simulink model "Robo_Bipede_Contato"  (R2020a)
settings: Solver=ode15s  StartTime=0.0  StopTime=1  MaxStep=1e-4  RelTol=1e-4  AbsTol=1e-5  EnableMultiTasking=on
model workspace: external: MATLAB File C:\Users\LUIS IZQUIERDO C\Desktop\PROGRAMAS TESE\13. ROBO BIPEDE SIMSCAPE COM CONTATO\Model_Params_Contato.m (data not in the file)
values from neighbouring files (symbols this model uses):
  CoG_y = 0.091733    [Model_Params_Cont_FSM.m]
  height_plane = 0.025    [Model_Params_Cont_FSM.m]
  m_esfera = 1    [Model_Params_Cont_FSM.m]
  plane_height = height_plane    (= 0.025)    [Model_Params_Cont_FSM.m]
  plane_length = 50    [Model_Params_Cont_FSM.m]
  plane_width = 3    [Model_Params_Cont_FSM.m]
  temp = Dados_XY1_D(ciclo,1)    [Model_Params_Cont_FSM.m]
  velocidade = 1    [Model_Params_Cont_FSM.m]
  Xpq2_D = Xpq2_D'    [Model_Params_Cont_FSM.m]
  Xpq3_D = Xpq3_D'    [Model_Params_Cont_FSM.m]
  Ypq2_D = Ypq2_D'    [Model_Params_Cont_FSM.m]
  Ypq3_D = Ypq3_D'    [Model_Params_Cont_FSM.m]
undefined symbols (not defined in the file or in its folder): COXA, HAT, PE, PERNA, X, Y, Z
libraries: nesl_utility x70, sm_lib x61, simulink x1
(part 1 of 3)
settings Model: Creator=LUIS IZQUIERDO C  LastModifiedBy=LUIS IZQUIERDO C
settings DataIOCC: LimitDataPoints=on  ReturnWorkspaceOutputs=off  LoggingToFile=on
settings OptimizationCC: LifeSpan=inf
settings DebuggingCC: AllowSymbolicDim=off  SFUnexpectedBacktrackingDiag=warning  SFNoUnconditionalDefaultTransitionDiag=warning  SFExecutionAtInitializationDiag=none  ArithmeticOperatorsInVariantConditions=warning
settings SFSimCC: SimUseLocalCustomCode=off  CustomCodeUndefinedFunction=UseInterfaceOnly
settings RTWCC: RTWUseLocalCustomCode=off
settings CodeAppCC: StateflowObjectComments=on
settings GRTTargetCC: TargetLangStandard=C89/C90 (ANSI)
settings ConfigComp: CovMetricSettings=dw  CovHtmlReporting=on  CovSaveCumulativeToWorkspaceVar=on  CovSaveSingleToWorkspaceVar=on  CovExternalEMLEnable=off  CovSFcnEnable=off
settings SimscapeCC: SimscapeNominalValues="[{\"value\":\"10\",\"unit\":\"V\"},{\"value\":\"1\",\"unit\":\"A\"},{\"value\":\"10\",\"unit\":\"N*m\"},{\"value\":\"10\",\"unit\":\"bar\"},{\"value\":\"100\",\"unit\":\"kJ/kg\"},{\"value\":\"1\",\"unit\":\"kW\"},{\"value\":\"300\",\"unit\":\"K\"},{\"value\":\"100\",\"unit\":\"cm^3/s\"},{\"value\":\"1\",\"unit\":\"kN\"},{\"value\":\"1\",\"unit\":\"g/cm^3\"},{\"value\":\"1\",\"unit\":\"l\"},{\"value\":\"1\",\"unit\":\"cm^2\"},{\"value\":\"60\",\"unit\":\"Hz\"}]"  SimscapeLogType=all  SimscapeLogDataHistory=10000
settings ConfigurationSet: Description=SimMechanics 2G

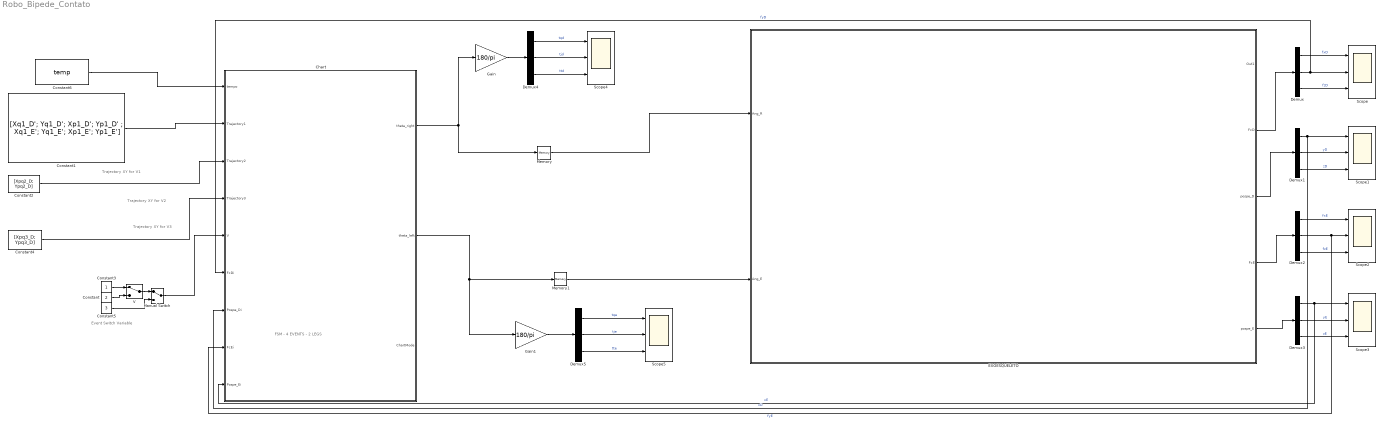
== system Robo_Bipede_Contato ==
  note: Trajectory XY for V1
  note: FSM - 4 EVENTS - 2 LEGS
  note: Trajectory XY for V2
  note: Trajectory XY for V3
  note: Event Switch Variable
  Chart : Stateflow chart  TreatAsAtomicUnit=on
  Constant : Constant  Value=2
  Constant1 : Constant  Value=|  VectorParams1D=off
      | [Xq1_D'; Yq1_D'; Xp1_D';
      | Yp1_D'
      | ;  Xq1_E';
      | Yq1_E';
      | Xp1_E';
      | Yp1_E']
  Constant2 : Constant  Value=[Xpq2_D; Ypq2_D]  VectorParams1D=off
  Constant3 : Constant
  Constant4 : Constant  Value=[Xpq3_D; Ypq3_D]  VectorParams1D=off
  Constant5 : Constant  Value=3
  Constant6 : Constant  Value=temp  VectorParams1D=off
  Demux{,1..5} (6 alike) : Demux  Outputs=3
  EXOESQUELETO : Subsystem
  Gain : Gain  Gain=180/pi
  Gain1 : Gain  Gain=180/pi
  Manual Switch : ManualSwitch
  Memory : Memory
  Memory1 : Memory
  Scope{,1..5} (6 alike) : Scope  NumInputPorts=3
  V : ManualSwitch
  wires:
  EXOESQUELETO/5(pospe_E) -> Demux3/1
  EXOESQUELETO/2(FcD) -> Demux/1
  Demux/1 -> Scope/1  "fxD"
  Demux/2 -> Chart/6(FcDi), Scope/2  "fyD"
  Demux/3 -> Scope/3  "fzD"
  Demux1/1 -> Chart/7(Pospe_Di), Scope1/1  "xD"
  Demux1/2 -> Scope1/2  "yD"
  Demux1/3 -> Scope1/3  "zD"
  Demux3/1 -> Chart/9(Pospe_Ei), Scope3/1  "xE"
  Demux3/2 -> Scope3/2  "yE"
  Demux2/1 -> Scope2/1  "fxE"
  Demux2/2 -> Chart/8(FcEi), Scope2/2  "fyE"
  Demux2/3 -> Scope2/3  "fzE"
  Demux3/3 -> Scope3/3  "zE"
  EXOESQUELETO/3(pospe_D) -> Demux1/1
  EXOESQUELETO/4(FcE) -> Demux2/1
  Constant3/1 -> V/1
  V/1 -> Manual Switch/1
  Manual Switch/1 -> Chart/5(V)
  Constant2/1 -> Chart/3(Trajectory2)
  Constant/1 -> V/2
  Constant4/1 -> Chart/4(Trajectory3)
  Constant5/1 -> Manual Switch/2
  Constant1/1 -> Chart/2(Trajectory1)
  Constant6/1 -> Chart/1(tempo)
  Chart/1(theta_right) -> Memory/1, Gain/1
  Memory/1 -> EXOESQUELETO/1(Ang_R)
  Memory1/1 -> EXOESQUELETO/2(Ang_E)
  Chart/2(theta_left) -> Gain1/1, Memory1/1
  Demux5/1 -> Scope5/1  "tqe"
  Demux5/2 -> Scope5/2  "tje"
  Demux5/3 -> Scope5/3  "tte"
  Demux4/2 -> Scope4/2  "tjd"
  Demux4/1 -> Scope4/1  "tqd"
  Demux4/3 -> Scope4/3  "ttd"
  Gain/1 -> Demux4/1
  Gain1/1 -> Demux5/1

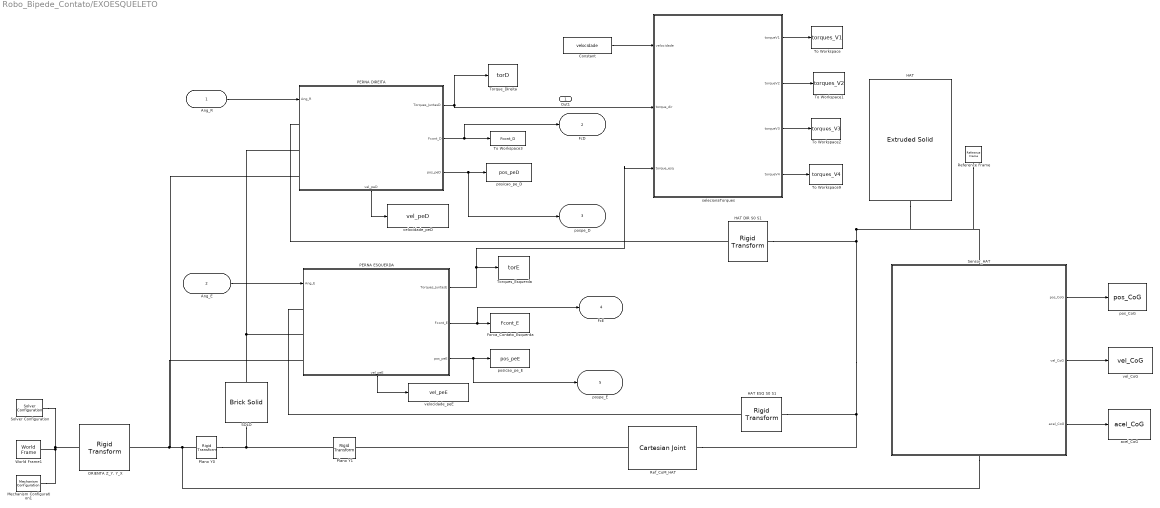
== system Robo_Bipede_Contato/EXOESQUELETO ==
  Ang_R : Inport
  Ang_E : Inport  Port=2
  Constant : Constant  Value=velocidade
  Forca_Contato_Esquerda : ToWorkspace  VariableName=Fcont_E  SaveFormat=Timeseries  SampleTime=-1
  HAT : sm_lib/Body Elements/Extruded Solid  GraphicAmbientColor=[0.15 0.15 0.15 1.0]  BasedOnType=Density  CenterOfMass=[0 0 0]  CenterOfMassUnits=m  GraphicDiffuseColor=[0.9 0.5 0.5]  ExportConvexHullGeometry=off  ExtrusionCrossSection=hat_cross_sec  ExtrusionCrossSectionUnits=m  Density=rho_ABS  DensityUnits=kg/m^3  DoExposeReferenceFrame=off  GraphicEmissiveColor=[0.0 0.0 0.0 1.0]  ExportEntireGeometry=off  ExtrusionLength=HAT.Profundidade  ExtrusionLengthUnits=m  ExtrusionType=General  SerializedFrames=<Frames><Frame><Id>Frame1</Id><Value><Name>CoG</Name><Origin><Source>CenterOfMassFrame</Source><FeatureName></FeatureName></Origin><PrimaryAxis><DefinedDirection>+Y</DefinedDirection><Source>CenterOfMassFrame</Source><SourceDirection>+Y</SourceDirection><FeatureName></FeatureName></PrimaryAxis><SecondaryAxis><DefinedDirection>+X</DefinedDirection><Source>CenterOfMassFrame</Source><SourceDirection>+Z</SourceDirection><FeatureName></FeatureName></SecondaryAxis></Value></Frame></Frames>  MarkerShape=Sphere  MarkerSize=10  GraphicType=FromGeometry  InertiaType=CalculateFromGeometry  Mass=HAT.Massa  MassUnits=kg  MomentsOfInertia=[1 1 1]  MomentsOfInertiaUnits=kg*m^2  PolygonNumSides=3  GraphicOpacity=1.0  PolygonOuterRadius=1  PolygonOuterRadiusUnits=m  ProductsOfInertia=[0 0 0]  ProductsOfInertiaUnits=kg*m^2  GraphicShininess=75  GraphicSpecularColor=[0.5 0.5 0.5 1.0]  GraphicVisPropType=SimpleVisualProperties
  HAT DIR S0 S1 : sm_lib/Frames and Transforms/Rigid Transform  TranslationMethod=Cartesian  TranslationStandardOffset=0  TranslationLengthUnit=m  TranslationStandardAxis=+Z  TranslationCartesianOffset="[0, -CoG_y,  HAT.Largura/2]"  TranslationROffset=0  TranslationROffsetUnits=m  TranslationZOffset=0  TranslationZOffsetUnits=m  TranslationThetaOffset=0  TranslationThetaOffsetUnits=deg  RotationMethod=None  RotationAngleUnits=deg  RotationStandardAxis=+Z  RotationAngle=0.0  RotationArbitraryAxis=[0 0 1]  FollAlignAxisA=+X  BaseAlignAxisA=+Y  FollAlignAxisB=+Y  BaseAlignAxisB=+Z  RotationSequenceAxes=FollowerAxes  RotationSequence=XYX  RotationSequenceAngles=[0 0 0]  RotationSequenceAnglesUnits=deg  RotationMatrix=[1 0 0; 0 1 0; 0 0 1]
  HAT ESQ S0 S1 : sm_lib/Frames and Transforms/Rigid Transform  TranslationMethod=Cartesian  TranslationStandardOffset=0  TranslationLengthUnit=m  TranslationStandardAxis=+Z  TranslationCartesianOffset="[0, -CoG_y,  -HAT.Largura/2]"  TranslationROffset=0  TranslationROffsetUnits=m  TranslationZOffset=0  TranslationZOffsetUnits=m  TranslationThetaOffset=0  TranslationThetaOffsetUnits=deg  RotationMethod=None  RotationAngleUnits=deg  RotationStandardAxis=+Z  RotationAngle=0.0  RotationArbitraryAxis=[0 0 1]  FollAlignAxisA=+X  BaseAlignAxisA=+Y  FollAlignAxisB=+Y  BaseAlignAxisB=+Z  RotationSequenceAxes=FollowerAxes  RotationSequence=XYX  RotationSequenceAngles=[0 0 0]  RotationSequenceAnglesUnits=deg  RotationMatrix=[1 0 0; 0 1 0; 0 0 1]
  Mechanism Configuration1 : sm_lib/Utilities/Mechanism Configuration  UniformGravity=Constant  GravityVector="[0, 0, -9.80665  ]"  GravityUnits=m/s^2  LinearizationDelta=0.001
  "ORIENTA Z_Y, Y_X " : sm_lib/Frames and Transforms/Rigid Transform  TranslationMethod=None  TranslationStandardOffset=0  TranslationLengthUnit=m  TranslationStandardAxis=+Z  TranslationCartesianOffset=[0 0 0]  TranslationROffset=0  TranslationROffsetUnits=m  TranslationZOffset=0  TranslationZOffsetUnits=m  TranslationThetaOffset=0  TranslationThetaOffsetUnits=deg  RotationMethod=AlignedAxes  RotationAngleUnits=deg  RotationStandardAxis=+Z  RotationAngle=0.0  RotationArbitraryAxis=[0 0 1]  FollAlignAxisA=+Y  BaseAlignAxisA=+Z  FollAlignAxisB=+X  BaseAlignAxisB=+Y  RotationSequenceAxes=FollowerAxes  RotationSequence=XYX  RotationSequenceAngles=[0 0 0]  RotationSequenceAnglesUnits=deg  RotationMatrix=[1 0 0; 0 1 0; 0 0 1]
  PERNA DIREITA : Subsystem
      settings: PortSchema="{\"entries\":[{\"content\":{\"sides\":[{\"content\":{\"connectorIds\":[\"In1\",\"LConn1\",\"LConn2\",\"LConn3\"]},\"type\":\"ConnectorPlacement.EquallySpacedRectSide\",\"uuid\":\"cc7b771d-19b2-48a5-9b25-497eb2125d6a\"},{\"content\":{\"connectorIds\":[\"Out1\",\"Out2\",\"Out3\"],\"side\":\"RIGHT\"},\"type\":\"ConnectorPlacement.EquallySpacedRectSide\",\"uuid\":\"a76f2280-f57a-4bff-8789-f2695d488ae9\"},{\"content\":{\"connectorIds\":[],\"side\":\"TOP\"},\"type\":\"ConnectorPlacement.EquallySpacedRectSide\",\"uuid\":\"65c05dcd-433d-4d8c-b019-0656464b6d1d\"},{\"content\":{\"connectorIds\":[\"Out4\"],\"side\":\"BOTTOM\"},\"type\":\"ConnectorPlacement.EquallySpacedRectSide\",\"uuid\":\"da520478-eb90-4d51-a918-9a7423737d50\"}]},\"type\":\"ConnectorPlacement.EquallySpacedConnector\",\"uuid\":\"0c78c314-db55-406a-a70d-77132cc9a0df\"}],\"packageUris\":[\"http://schema.mathworks.com/mf0/Connector/19700101\"],\"version\":\"1.0\"}"
  PERNA ESQUERDA : Subsystem
      settings: PortSchema="{\"entries\":[{\"content\":{\"sides\":[{\"content\":{\"connectorIds\":[\"In1\",\"LConn1\",\"LConn2\",\"LConn3\"]},\"type\":\"ConnectorPlacement.EquallySpacedRectSide\",\"uuid\":\"cc7b771d-19b2-48a5-9b25-497eb2125d6a\"},{\"content\":{\"connectorIds\":[\"Out1\",\"Out2\",\"Out3\"],\"side\":\"RIGHT\"},\"type\":\"ConnectorPlacement.EquallySpacedRectSide\",\"uuid\":\"a76f2280-f57a-4bff-8789-f2695d488ae9\"},{\"content\":{\"connectorIds\":[],\"side\":\"TOP\"},\"type\":\"ConnectorPlacement.EquallySpacedRectSide\",\"uuid\":\"65c05dcd-433d-4d8c-b019-0656464b6d1d\"},{\"content\":{\"connectorIds\":[\"Out4\"],\"side\":\"BOTTOM\"},\"type\":\"ConnectorPlacement.EquallySpacedRectSide\",\"uuid\":\"d42ce1bf-fe8c-427b-9e44-082b543e9a23\"}]},\"type\":\"ConnectorPlacement.EquallySpacedConnector\",\"uuid\":\"0c78c314-db55-406a-a70d-77132cc9a0df\"}],\"packageUris\":[\"http://schema.mathworks.com/mf0/Connector/19700101\"],\"version\":\"1.0\"}"
  "Plano Y0 " : sm_lib/Frames and Transforms/Rigid Transform  TranslationMethod=StandardAxis  TranslationStandardOffset=height_plane/2  TranslationLengthUnit=m  TranslationStandardAxis=-Y  TranslationCartesianOffset=[0 0 0]  TranslationROffset=0  TranslationROffsetUnits=m  TranslationZOffset=0  TranslationZOffsetUnits=m  TranslationThetaOffset=0  TranslationThetaOffsetUnits=deg  RotationMethod=StandardAxis  RotationAngleUnits=deg  RotationStandardAxis=+Z  RotationAngle=0  RotationArbitraryAxis=[0 0 1]  FollAlignAxisA=+X  BaseAlignAxisA=+Y  FollAlignAxisB=+Y  BaseAlignAxisB=+Z  RotationSequenceAxes=FollowerAxes  RotationSequence=XYX  RotationSequenceAngles=[0 0 0]  RotationSequenceAnglesUnits=deg  RotationMatrix=[1 0 0; 0 1 0; 0 0 1]
  Plano Y1 : sm_lib/Frames and Transforms/Rigid Transform  TranslationMethod=StandardAxis  TranslationStandardOffset=height_plane/2  TranslationLengthUnit=m  TranslationStandardAxis=+Y  TranslationCartesianOffset=[0 0 0]  TranslationROffset=0  TranslationROffsetUnits=m  TranslationZOffset=0  TranslationZOffsetUnits=m  TranslationThetaOffset=0  TranslationThetaOffsetUnits=deg  RotationMethod=None  RotationAngleUnits=deg  RotationStandardAxis=+Z  RotationAngle=0.0  RotationArbitraryAxis=[0 0 1]  FollAlignAxisA=+X  BaseAlignAxisA=+Y  FollAlignAxisB=+Y  BaseAlignAxisB=+Z  RotationSequenceAxes=FollowerAxes  RotationSequence=XYX  RotationSequenceAngles=[0 0 0]  RotationSequenceAnglesUnits=deg  RotationMatrix=[1 0 0; 0 1 0; 0 0 1]
  Ref_CoM_HAT : sm_lib/Joints/Cartesian Joint  JointMode=Normal  SenseConstraintForce=off  SenseConstraintForceX=off  SenseConstraintForceY=off  SenseConstraintForceZ=off  SenseConstraintTorque=off  SenseConstraintTorqueX=off  SenseConstraintTorqueY=off  SenseConstraintTorqueZ=off  SenseTotalForce=off  SenseTotalForceX=off  SenseTotalForceY=off  SenseTotalForceZ=off  SenseTotalTorque=off  SenseTotalTorqueX=off  SenseTotalTorqueY=off  SenseTotalTorqueZ=off  CompositeWrenchDir=FollowerOnBase  CompositeWrenchFrame=BaseFrame  PxEquilibriumPosition=0  PxEquilibriumPositionUnits=m  PxSpringStiffness=0  PxSpringStiffnessUnits=N/m  PxDampingCoefficient=0  PxDampingCoefficientUnits=N/(m/s)  PxTorqueActuationMode=NoTorque  PxMotionActuationMode=ComputedMotion  PxSensePosition=off  PxSenseVelocity=off  PxSenseAcceleration=off  PxSenseTorqueForce=off  PxSenseLowerLimitTorqueForce=off  PxSenseUpperLimitTorqueForce=off  PxLowerLimitSpecify=off  PxLowerLimitBound=-1  PxLowerLimitBoundUnits=m  PxLowerLimitStiffness=1e6  PxLowerLimitStiffnessUnits=N/m  PxLowerLimitDamping=1e3  PxLowerLimitDampingUnits=N/(m/s)  PxLowerLimitTransitionRegionWidth=1e-4  PxLowerLimitTransitionRegionWidthUnits=m  PxUpperLimitSpecify=off  PxUpperLimitBound=1  PxUpperLimitBoundUnits=m  PxUpperLimitStiffness=1e6  PxUpperLimitStiffnessUnits=N/m  PxUpperLimitDamping=1e3  PxUpperLimitDampingUnits=N/(m/s)  PxUpperLimitTransitionRegionWidth=1e-4  PxUpperLimitTransitionRegionWidthUnits=m  PxPositionTargetSpecify=off  PxPositionTargetPriority=High  PxPositionTargetValue=0  PxPositionTargetValueUnits=m  PxVelocityTargetSpecify=off  PxVelocityTargetPriority=High  PxVelocityTargetValue=0  PxVelocityTargetValueUnits=m/s  PyEquilibriumPosition=0  PyEquilibriumPositionUnits=m  PySpringStiffness=0  PySpringStiffnessUnits=N/m  PyDampingCoefficient=0  PyDampingCoefficientUnits=N/(m/s)  PyTorqueActuationMode=NoTorque  PyMotionActuationMode=ComputedMotion  PySensePosition=off  PySenseVelocity=off  PySenseAcceleration=off  PySenseTorqueForce=off  PySenseLowerLimitTorqueForce=off  PySenseUpperLimitTorqueForce=off  PyLowerLimitSpecify=off  PyLowerLimitBound=-1  PyLowerLimitBoundUnits=m  PyLowerLimitStiffness=1e6  PyLowerLimitStiffnessUnits=N/m  PyLowerLimitDamping=1e3  PyLowerLimitDampingUnits=N/(m/s)  PyLowerLimitTransitionRegionWidth=1e-4  PyLowerLimitTransitionRegionWidthUnits=m  PyUpperLimitSpecify=off  PyUpperLimitBound=1  PyUpperLimitBoundUnits=m  PyUpperLimitStiffness=1e6  PyUpperLimitStiffnessUnits=N/m  PyUpperLimitDamping=1e3  PyUpperLimitDampingUnits=N/(m/s)  PyUpperLimitTransitionRegionWidth=1e-4  PyUpperLimitTransitionRegionWidthUnits=m  PyPositionTargetSpecify=on  PyPositionTargetPriority=High  PyPositionTargetValue=hat_alt_ini  PyPositionTargetValueUnits=m  PyVelocityTargetSpecify=off  PyVelocityTargetPriority=High  PyVelocityTargetValue=0  PyVelocityTargetValueUnits=m/s  PzEquilibriumPosition=0  PzEquilibriumPositionUnits=m  PzSpringStiffness=0  PzSpringStiffnessUnits=N/m  PzDampingCoefficient=0  PzDampingCoefficientUnits=N/(m/s)  PzTorqueActuationMode=NoTorque  PzMotionActuationMode=ComputedMotion  PzSensePosition=off  PzSenseVelocity=off  PzSenseAcceleration=off  PzSenseTorqueForce=off  PzSenseLowerLimitTorqueForce=off  PzSenseUpperLimitTorqueForce=off  PzLowerLimitSpecify=off  PzLowerLimitBound=-1  PzLowerLimitBoundUnits=m  PzLowerLimitStiffness=1e6  PzLowerLimitStiffnessUnits=N/m  PzLowerLimitDamping=1e3  PzLowerLimitDampingUnits=N/(m/s)  PzLowerLimitTransitionRegionWidth=1e-4  PzLowerLimitTransitionRegionWidthUnits=m  PzUpperLimitSpecify=off  PzUpperLimitBound=1  PzUpperLimitBoundUnits=m  PzUpperLimitStiffness=1e6  PzUpperLimitStiffnessUnits=N/m  PzUpperLimitDamping=1e3  PzUpperLimitDampingUnits=N/(m/s)  PzUpperLimitTransitionRegionWidth=1e-4  PzUpperLimitTransitionRegionWidthUnits=m  PzPositionTargetSpecify=off  PzPositionTargetPriority=High  PzPositionTargetValue=0  PzPositionTargetValueUnits=m  PzVelocityTargetSpecify=off  PzVelocityTargetPriority=High  PzVelocityTargetValue=0  PzVelocityTargetValueUnits=m/s
  Reference Frame : sm_lib/Frames and Transforms/Reference Frame
  "SOLO " : sm_lib/Body Elements/Brick Solid  GraphicAmbientColor=[0.15 0.15 0.15 1.0]  BasedOnType=Density  BrickDimensions=[plane_length plane_height plane_width]  BrickDimensionUnits=m  CenterOfMass=[0 0 0]  CenterOfMassUnits=m  GraphicDiffuseColor=[0.0 0.6 0.6]  Density=rho_solo  DensityUnits=kg/m^3  DoExposeReferenceFrame=on  GraphicEmissiveColor=[0.0 0.0 0.0 1.0]  ExportEntireGeometry=on  SerializedFrames=<Frames/>  MarkerShape=Sphere  MarkerSize=10  GraphicType=FromGeometry  InertiaType=CalculateFromGeometry  Mass=1  MassUnits=kg  MomentsOfInertia=[1 1 1]  MomentsOfInertiaUnits=kg*m^2  GraphicOpacity=0.4  ProductsOfInertia=[0 0 0]  ProductsOfInertiaUnits=kg*m^2  GraphicShininess=10  GraphicSpecularColor=[0.5 0.5 0.5 1.0]  GraphicVisPropType=AdvancedVisualProperties
  Sensor_HAT : Subsystem
      settings: PortSchema="{\"entries\":[{\"content\":{\"sides\":[{\"content\":{\"connectorIds\":[]},\"type\":\"ConnectorPlacement.EquallySpacedRectSide\",\"uuid\":\"769ee7b6-bdc6-49d9-8637-a9c81876e313\"},{\"content\":{\"connectorIds\":[\"Out1\",\"Out2\",\"Out3\"],\"side\":\"RIGHT\"},\"type\":\"ConnectorPlacement.EquallySpacedRectSide\",\"uuid\":\"1964de58-24b6-444a-bc2a-64d941588411\"},{\"content\":{\"connectorIds\":[\"LConn1\"],\"side\":\"TOP\"},\"type\":\"ConnectorPlacement.EquallySpacedRectSide\",\"uuid\":\"8b94c6c7-97d0-4ec3-af06-f5ebe0bb7cbe\"},{\"content\":{\"connectorIds\":[\"RConn1\"],\"side\":\"BOTTOM\"},\"type\":\"ConnectorPlacement.EquallySpacedRectSide\",\"uuid\":\"865a678d-12ed-4989-bf96-8b8e46d0c823\"}]},\"type\":\"ConnectorPlacement.EquallySpacedConnector\",\"uuid\":\"6708977a-50fa-47ad-9803-8cc7bd37c0d7\"}],\"packageUris\":[\"http://schema.mathworks.com/mf0/Connector/19700101\"],\"version\":\"1.0\"}"
  Solver Configuration : nesl_utility/Solver Configuration  PhysicalDomain=network_engine_domain  SubClassName=solver  LeftPortType=input  RightPortType=generic  Tones=[]  Harmonics=[]  SimulateNoise=off  Profile=off  UseLocalSampling=off  EnableSwitchedLinearOptims=on  FrequencyDomain=off  UseCCode=off  RelTol=0.001  AbsTol=1e-06  MinStep=1e-09  ToWorkspace=off  RevertToSquareIcSolve=off  NumHomotopyIterations=100  PhasorMode=off  PhasorModeNumHarmonics=1  DoDC=off  ResidualTolerance=1e-09  UseLocalSolver=off  LocalSolverChoice=NE_BACKWARD_EULER_ADVANCER  LocalSolverSampleTime=0.001  DoFixedCost=off  MaxNonlinIter=3  MaxModeIter=2  LinearAlgebra=Sparse  EquationFormulation=NE_TIME_EF  DelaysMemoryBudget=1024  AutomaticFiltering=on  FilteringTimeConstant=0.001  PartitionStorageMethod=AS_NEEDED  PartitionMemoryBudget=1024  PartitionMethod=FAST
  To Workspace : ToWorkspace  VariableName=torques_V1  SaveFormat=Timeseries  SampleTime=-1
  To Workspace1 : ToWorkspace  VariableName=torques_V2  SaveFormat=Timeseries  SampleTime=-1
  To Workspace2 : ToWorkspace  VariableName=torques_V3  SaveFormat=Timeseries  SampleTime=-1
  To Workspace3 : ToWorkspace  VariableName=Fcont_D  SaveFormat=Timeseries  SampleTime=-1
  To Workspace9 : ToWorkspace  VariableName=torques_V4  SaveFormat=Timeseries  SampleTime=-1
  Torque_Direita : ToWorkspace  VariableName=torD  SaveFormat=Timeseries  SampleTime=-1
  Torques_Esquerda : ToWorkspace  VariableName=torE  SaveFormat=Timeseries  SampleTime=-1
  World Frame1 : sm_lib/Frames and Transforms/World Frame
  acel_CoG : ToWorkspace  VariableName=acel_CoG  SaveFormat=Timeseries  SampleTime=-1
  pos_CoG : ToWorkspace  VariableName=pos_CoG  SaveFormat=Timeseries  SampleTime=-1
  posicao_pe_D : ToWorkspace  VariableName=pos_peD  SaveFormat=Timeseries  SampleTime=-1
  posicao_pe_E : ToWorkspace  VariableName=pos_peE  SaveFormat=Timeseries  SampleTime=-1
  selecionaTorques : MATLAB Function  TreatAsAtomicUnit=on
  vel_CoG : ToWorkspace  VariableName=vel_CoG  SaveFormat=Timeseries  SampleTime=-1
  velocidade_peD : ToWorkspace  VariableName=vel_peD  SaveFormat=Timeseries  SampleTime=-1
  velocidade_peE : ToWorkspace  VariableName=vel_peE  SaveFormat=Timeseries  SampleTime=-1
  Out1 : Outport
  FcD : Outport  Port=2
  pospe_D : Outport  Port=3
  FcE : Outport  Port=4
  pospe_E : Outport  Port=5
  wires:
  PERNA ESQUERDA/1("Torques_JuntasE ") -> Torques_Esquerda/1, selecionaTorques/3(torque_esq)
  Ang_R/1 -> PERNA DIREITA/1(Ang_R)
  PERNA DIREITA/1("Torques_JuntasD ") -> Torque_Direita/1, selecionaTorques/2(torque_dir)
  selecionaTorques/2(torqueV2) -> To Workspace1/1
  selecionaTorques/3(torqueV3) -> To Workspace2/1
  Sensor_HAT/1(pos_CoG) -> pos_CoG/1
  PERNA ESQUERDA/2(Fcont_E) -> FcE/1, Forca_Contato_Esquerda/1
  Ang_E/1 -> PERNA ESQUERDA/1(Ang_E)
  Sensor_HAT/2(vel_CoG) -> vel_CoG/1
  selecionaTorques/4(torqueV4) -> To Workspace9/1
  Sensor_HAT/3(acel_CoG) -> acel_CoG/1
  PERNA ESQUERDA/3(pos_peE) -> pospe_E/1, posicao_pe_E/1
  PERNA DIREITA/2(Fcont_D) -> To Workspace3/1, FcD/1
  PERNA ESQUERDA/4(vel_peE) -> velocidade_peE/1
  selecionaTorques/1(torqueV1) -> To Workspace/1
  Constant/1 -> selecionaTorques/1(velocidade)
  PERNA DIREITA/3(pos_peD) -> posicao_pe_D/1, pospe_D/1
  PERNA DIREITA/4(vel_peD) -> velocidade_peD/1
  connections:
  PERNA DIREITA/LConn1 -- HAT DIR S0 S1/RConn1
  PERNA ESQUERDA/LConn1 -- HAT ESQ S0 S1/RConn1
  Ref_CoM_HAT/LConn1 -- Plano Y1/RConn1
  "Plano Y0 "/RConn1 -- PERNA DIREITA/LConn3 -- PERNA ESQUERDA/LConn3 -- "ORIENTA Z_Y, Y_X "/RConn1 -- Sensor_HAT/RConn1
  Ref_CoM_HAT/RConn1 -- Reference Frame/RConn1 -- HAT/LConn1 -- Sensor_HAT/LConn1 -- HAT DIR S0 S1/LConn1 -- HAT ESQ S0 S1/LConn1
  "SOLO "/RConn1 -- "Plano Y0 "/LConn1 -- Plano Y1/LConn1
  "SOLO "/LConn1 -- PERNA DIREITA/LConn2 -- PERNA ESQUERDA/LConn2
  Solver Configuration/RConn1 -- "ORIENTA Z_Y, Y_X "/LConn1 -- Mechanism Configuration1/RConn1 -- World Frame1/RConn1

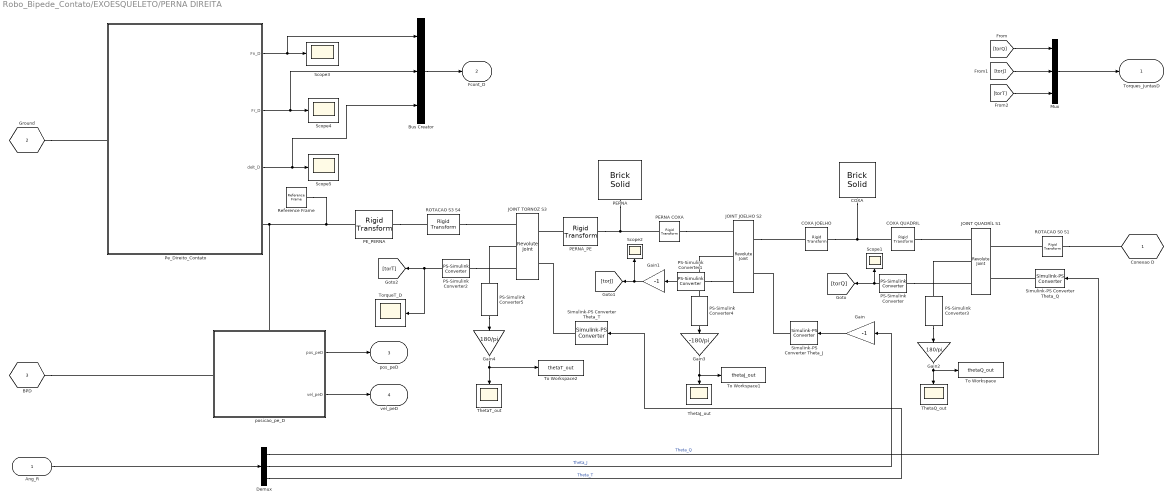
== system Robo_Bipede_Contato/EXOESQUELETO/PERNA DIREITA ==
  Ang_R : Inport
  Bus Creator : BusCreator  Inputs=3
  COXA : sm_lib/Body Elements/Brick Solid  GraphicAmbientColor=[0.15 0.15 0.15 1.0]  BasedOnType=Density  BrickDimensions="[COXA.Comprimento,  COXA.Profundidade,  COXA.Largura]"  BrickDimensionUnits=m  CenterOfMass=[0 0 0]  CenterOfMassUnits=m  GraphicDiffuseColor=cor_coxa  Density=rho_ABS  DensityUnits=kg/m^3  DoExposeReferenceFrame=on  GraphicEmissiveColor=[0.0 0.0 0.0 1.0]  ExportEntireGeometry=off  SerializedFrames=<Frames/>  MarkerShape=Sphere  MarkerSize=10  GraphicType=FromGeometry  InertiaType=CalculateFromGeometry  Mass=1  MassUnits=kg  MomentsOfInertia=[1 1 1]  MomentsOfInertiaUnits=kg*m^2  GraphicOpacity=1.0  ProductsOfInertia=[0 0 0]  ProductsOfInertiaUnits=kg*m^2  GraphicShininess=75  GraphicSpecularColor=[0.5 0.5 0.5 1.0]  GraphicVisPropType=SimpleVisualProperties
  COXA JOELHO : sm_lib/Frames and Transforms/Rigid Transform  TranslationMethod=StandardAxis  TranslationStandardOffset=COXA.Comprimento/2  TranslationLengthUnit=m  TranslationStandardAxis=+X  TranslationCartesianOffset=[0 0 0]  TranslationROffset=0  TranslationROffsetUnits=m  TranslationZOffset=0  TranslationZOffsetUnits=m  TranslationThetaOffset=0  TranslationThetaOffsetUnits=deg  RotationMethod=None  RotationAngleUnits=deg  RotationStandardAxis=+Z  RotationAngle=0.0  RotationArbitraryAxis=[0 0 1]  FollAlignAxisA=+X  BaseAlignAxisA=+Y  FollAlignAxisB=+Y  BaseAlignAxisB=+Z  RotationSequenceAxes=FollowerAxes  RotationSequence=XYX  RotationSequenceAngles=[0 0 0]  RotationSequenceAnglesUnits=deg  RotationMatrix=[1 0 0; 0 1 0; 0 0 1]
  COXA QUADRIL : sm_lib/Frames and Transforms/Rigid Transform  TranslationMethod=StandardAxis  TranslationStandardOffset=COXA.Comprimento/2  TranslationLengthUnit=m  TranslationStandardAxis=-X  TranslationCartesianOffset=[0 0 0]  TranslationROffset=0  TranslationROffsetUnits=m  TranslationZOffset=0  TranslationZOffsetUnits=m  TranslationThetaOffset=0  TranslationThetaOffsetUnits=deg  RotationMethod=None  RotationAngleUnits=deg  RotationStandardAxis=+Z  RotationAngle=0.0  RotationArbitraryAxis=[0 0 1]  FollAlignAxisA=+X  BaseAlignAxisA=+Y  FollAlignAxisB=+Y  BaseAlignAxisB=+Z  RotationSequenceAxes=FollowerAxes  RotationSequence=XYX  RotationSequenceAngles=[0 0 0]  RotationSequenceAnglesUnits=deg  RotationMatrix=[1 0 0; 0 1 0; 0 0 1]
  Demux : Demux  Outputs=3
  Gain : Gain  Gain=-1
  Gain1 : Gain  Gain=-1
  Gain2 : Gain  Gain=180/pi
  Gain3 : Gain  Gain=-180/pi
  Gain4 : Gain  Gain=180/pi
  JOINT JOELHO S2 : sm_lib/Joints/Revolute Joint  JointMode=Normal  SenseConstraintForce=off  SenseConstraintForceX=off  SenseConstraintForceY=off  SenseConstraintForceZ=off  SenseConstraintTorque=off  SenseConstraintTorqueX=off  SenseConstraintTorqueY=off  SenseConstraintTorqueZ=off  SenseTotalForce=off  SenseTotalForceX=off  SenseTotalForceY=off  SenseTotalForceZ=off  SenseTotalTorque=off  SenseTotalTorqueX=off  SenseTotalTorqueY=off  SenseTotalTorqueZ=off  CompositeWrenchDir=FollowerOnBase  CompositeWrenchFrame=BaseFrame  EquilibriumPosition=0  EquilibriumPositionUnits=rad  SpringStiffness=0  SpringStiffnessUnits=N*m/rad  DampingCoefficient=Damping_junta  DampingCoefficientUnits=N*m/(rad/s)  TorqueActuationMode=ComputedTorque  MotionActuationMode=InputMotion  SensePosition=on  SenseVelocity=off  SenseAcceleration=off  SenseTorqueForce=on  SenseLowerLimitTorqueForce=off  SenseUpperLimitTorqueForce=off  LowerLimitSpecify=off  LowerLimitBound=-90  LowerLimitBoundUnits=deg  LowerLimitStiffness=1e4  LowerLimitStiffnessUnits=N*m/deg  LowerLimitDamping=10  LowerLimitDampingUnits=N*m/(deg/s)  LowerLimitTransitionRegionWidth=0.1  LowerLimitTransitionRegionWidthUnits=deg  UpperLimitSpecify=off  UpperLimitBound=90  UpperLimitBoundUnits=deg  UpperLimitStiffness=1e4  UpperLimitStiffnessUnits=N*m/deg  UpperLimitDamping=10  UpperLimitDampingUnits=N*m/(deg/s)  UpperLimitTransitionRegionWidth=0.1  UpperLimitTransitionRegionWidthUnits=deg  PositionTargetSpecify=on  PositionTargetPriority=High  PositionTargetValue=thetaJ_D0  PositionTargetValueUnits=rad  VelocityTargetSpecify=off  VelocityTargetPriority=High  VelocityTargetValue=0  VelocityTargetValueUnits=deg/s
  JOINT QUADRlL S1 : sm_lib/Joints/Revolute Joint  JointMode=Normal  SenseConstraintForce=off  SenseConstraintForceX=off  SenseConstraintForceY=off  SenseConstraintForceZ=off  SenseConstraintTorque=off  SenseConstraintTorqueX=off  SenseConstraintTorqueY=off  SenseConstraintTorqueZ=off  SenseTotalForce=off  SenseTotalForceX=off  SenseTotalForceY=off  SenseTotalForceZ=off  SenseTotalTorque=off  SenseTotalTorqueX=off  SenseTotalTorqueY=off  SenseTotalTorqueZ=off  CompositeWrenchDir=FollowerOnBase  CompositeWrenchFrame=BaseFrame  EquilibriumPosition=0  EquilibriumPositionUnits=rad  SpringStiffness=0  SpringStiffnessUnits=N*m/rad  DampingCoefficient=Damping_junta  DampingCoefficientUnits=N*m/(rad/s)  TorqueActuationMode=ComputedTorque  MotionActuationMode=InputMotion  SensePosition=on  SenseVelocity=off  SenseAcceleration=off  SenseTorqueForce=on  SenseLowerLimitTorqueForce=off  SenseUpperLimitTorqueForce=off  LowerLimitSpecify=off  LowerLimitBound=-90  LowerLimitBoundUnits=deg  LowerLimitStiffness=1e4  LowerLimitStiffnessUnits=N*m/deg  LowerLimitDamping=10  LowerLimitDampingUnits=N*m/(deg/s)  LowerLimitTransitionRegionWidth=0.1  LowerLimitTransitionRegionWidthUnits=deg  UpperLimitSpecify=off  UpperLimitBound=90  UpperLimitBoundUnits=deg  UpperLimitStiffness=1e4  UpperLimitStiffnessUnits=N*m/deg  UpperLimitDamping=10  UpperLimitDampingUnits=N*m/(deg/s)  UpperLimitTransitionRegionWidth=0.1  UpperLimitTransitionRegionWidthUnits=deg  PositionTargetSpecify=on  PositionTargetPriority=High  PositionTargetValue=thetaQ_D0  PositionTargetValueUnits=rad  VelocityTargetSpecify=off  VelocityTargetPriority=High  VelocityTargetValue=0  VelocityTargetValueUnits=deg/s
  JOINT TORNOZ S3 : sm_lib/Joints/Revolute Joint  JointMode=Normal  SenseConstraintForce=off  SenseConstraintForceX=off  SenseConstraintForceY=off  SenseConstraintForceZ=off  SenseConstraintTorque=off  SenseConstraintTorqueX=off  SenseConstraintTorqueY=off  SenseConstraintTorqueZ=off  SenseTotalForce=off  SenseTotalForceX=off  SenseTotalForceY=off  SenseTotalForceZ=off  SenseTotalTorque=off  SenseTotalTorqueX=off  SenseTotalTorqueY=off  SenseTotalTorqueZ=off  CompositeWrenchDir=FollowerOnBase  CompositeWrenchFrame=BaseFrame  EquilibriumPosition=0  EquilibriumPositionUnits=rad  SpringStiffness=0  SpringStiffnessUnits=N*m/rad  DampingCoefficient=Damping_junta  DampingCoefficientUnits=N*m/(rad/s)  TorqueActuationMode=ComputedTorque  MotionActuationMode=InputMotion  SensePosition=on  SenseVelocity=off  SenseAcceleration=off  SenseTorqueForce=on  SenseLowerLimitTorqueForce=off  SenseUpperLimitTorqueForce=off  LowerLimitSpecify=off  LowerLimitBound=-90  LowerLimitBoundUnits=deg  LowerLimitStiffness=1e4  LowerLimitStiffnessUnits=N*m/deg  LowerLimitDamping=10  LowerLimitDampingUnits=N*m/(deg/s)  LowerLimitTransitionRegionWidth=0.1  LowerLimitTransitionRegionWidthUnits=deg  UpperLimitSpecify=off  UpperLimitBound=90  UpperLimitBoundUnits=deg  UpperLimitStiffness=1e4  UpperLimitStiffnessUnits=N*m/deg  UpperLimitDamping=10  UpperLimitDampingUnits=N*m/(deg/s)  UpperLimitTransitionRegionWidth=0.1  UpperLimitTransitionRegionWidthUnits=deg  PositionTargetSpecify=on  PositionTargetPriority=High  PositionTargetValue=thetaT_D0  PositionTargetValueUnits=rad  VelocityTargetSpecify=off  VelocityTargetPriority=High  VelocityTargetValue=0  VelocityTargetValueUnits=deg/s
  Mux : Mux  Inputs=3
  PERNA : sm_lib/Body Elements/Brick Solid  GraphicAmbientColor=[0.15 0.15 0.15 1.0]  BasedOnType=Density  BrickDimensions=[PERNA.Comprimento, PERNA.Profundidade, PERNA.Largura]  BrickDimensionUnits=m  CenterOfMass=[0 0 0]  CenterOfMassUnits=m  GraphicDiffuseColor=cor_perna  Density=rho_ABS  DensityUnits=kg/m^3  DoExposeReferenceFrame=on  GraphicEmissiveColor=[0.0 0.0 0.0 1.0]  ExportEntireGeometry=off  SerializedFrames=<Frames/>  MarkerShape=Sphere  MarkerSize=10  GraphicType=FromGeometry  InertiaType=CalculateFromGeometry  Mass=1  MassUnits=kg  MomentsOfInertia=[1 1 1]  MomentsOfInertiaUnits=kg*m^2  GraphicOpacity=1.0  ProductsOfInertia=[0 0 0]  ProductsOfInertiaUnits=kg*m^2  GraphicShininess=75  GraphicSpecularColor=[0.5 0.5 0.5 1.0]  GraphicVisPropType=SimpleVisualProperties
  PERNA COXA : sm_lib/Frames and Transforms/Rigid Transform  TranslationMethod=StandardAxis  TranslationStandardOffset=PERNA.Comprimento/2  TranslationLengthUnit=m  TranslationStandardAxis=-X  TranslationCartesianOffset=[0 0 0]  TranslationROffset=0  TranslationROffsetUnits=m  TranslationZOffset=0  TranslationZOffsetUnits=m  TranslationThetaOffset=0  TranslationThetaOffsetUnits=deg  RotationMethod=None  RotationAngleUnits=deg  RotationStandardAxis=+Z  RotationAngle=0.0  RotationArbitraryAxis=[0 0 1]  FollAlignAxisA=+X  BaseAlignAxisA=+Y  FollAlignAxisB=+Y  BaseAlignAxisB=+Z  RotationSequenceAxes=FollowerAxes  RotationSequence=XYX  RotationSequenceAngles=[0 0 0]  RotationSequenceAnglesUnits=deg  RotationMatrix=[1 0 0; 0 1 0; 0 0 1]
  PERNA_PE : sm_lib/Frames and Transforms/Rigid Transform  TranslationMethod=Cartesian  TranslationStandardOffset=0  TranslationLengthUnit=m  TranslationStandardAxis=+Z  TranslationCartesianOffset=[PERNA.Comprimento/2, -PERNA.Profundidade/2, 0]  TranslationROffset=0  TranslationROffsetUnits=m  TranslationZOffset=0  TranslationZOffsetUnits=m  TranslationThetaOffset=0  TranslationThetaOffsetUnits=deg  RotationMethod=None  RotationAngleUnits=deg  RotationStandardAxis=+Z  RotationAngle=0.0  RotationArbitraryAxis=[0 0 1]  FollAlignAxisA=+X  BaseAlignAxisA=+Y  FollAlignAxisB=+Y  BaseAlignAxisB=+Z  RotationSequenceAxes=FollowerAxes  RotationSequence=XYX  RotationSequenceAngles=[0 0 0]  RotationSequenceAnglesUnits=deg  RotationMatrix=[1 0 0; 0 1 0; 0 0 1]
  PE_PERNA : sm_lib/Frames and Transforms/Rigid Transform  TranslationMethod=Cartesian  TranslationStandardOffset=0  TranslationLengthUnit=m  TranslationStandardAxis=+Z  TranslationCartesianOffset=[-PE.Comprimento/2, 0, 0]  TranslationROffset=0  TranslationROffsetUnits=m  TranslationZOffset=0  TranslationZOffsetUnits=m  TranslationThetaOffset=0  TranslationThetaOffsetUnits=deg  RotationMethod=None  RotationAngleUnits=deg  RotationStandardAxis=+Z  RotationAngle=0.0  RotationArbitraryAxis=[0 0 1]  FollAlignAxisA=+X  BaseAlignAxisA=+Y  FollAlignAxisB=+Y  BaseAlignAxisB=+Z  RotationSequenceAxes=FollowerAxes  RotationSequence=XYX  RotationSequenceAngles=[0 0 0]  RotationSequenceAnglesUnits=deg  RotationMatrix=[1 0 0; 0 1 0; 0 0 1]
  PS-Simulink Converter : nesl_utility/PS-Simulink Converter  PhysicalDomain=network_engine_domain  SubClassName=ps_output  LeftPortType=input  RightPortType=output  PseudoPeriodic=off  Frequencies=[]  Unit=N*m  AffineConversion=off
  PS-Simulink Converter1 : nesl_utility/PS-Simulink Converter  PhysicalDomain=network_engine_domain  SubClassName=ps_output  LeftPortType=input  RightPortType=output  PseudoPeriodic=off  Frequencies=[]  Unit=N*m  AffineConversion=off
  PS-Simulink Converter{2..5} (4 alike) : nesl_utility/PS-Simulink Converter  PhysicalDomain=network_engine_domain  SubClassName=ps_output  LeftPortType=input  RightPortType=output  PseudoPeriodic=off  Frequencies=[]  Unit=1  AffineConversion=off
  Pe_Direito_Contato : Subsystem
  ROTACAO S0 S1 : sm_lib/Frames and Transforms/Rigid Transform  TranslationMethod=None  TranslationStandardOffset=0  TranslationLengthUnit=m  TranslationStandardAxis=+Z  TranslationCartesianOffset=[0 0 0]  TranslationROffset=0  TranslationROffsetUnits=m  TranslationZOffset=0  TranslationZOffsetUnits=m  TranslationThetaOffset=0  TranslationThetaOffsetUnits=deg  RotationMethod=StandardAxis  RotationAngleUnits=deg  RotationStandardAxis=+Z  RotationAngle=-90  RotationArbitraryAxis=[0 0 1]  FollAlignAxisA=+X  BaseAlignAxisA=+Y  FollAlignAxisB=+Y  BaseAlignAxisB=+Z  RotationSequenceAxes=FollowerAxes  RotationSequence=XYX  RotationSequenceAngles=[0 0 0]  RotationSequenceAnglesUnits=deg  RotationMatrix=[1 0 0; 0 1 0; 0 0 1]
  ROTACAO S3 S4 : sm_lib/Frames and Transforms/Rigid Transform  TranslationMethod=None  TranslationStandardOffset=0  TranslationLengthUnit=m  TranslationStandardAxis=+Z  TranslationCartesianOffset=[0 0 0]  TranslationROffset=0  TranslationROffsetUnits=m  TranslationZOffset=0  TranslationZOffsetUnits=m  TranslationThetaOffset=0  TranslationThetaOffsetUnits=deg  RotationMethod=StandardAxis  RotationAngleUnits=deg  RotationStandardAxis=+Z  RotationAngle=90  RotationArbitraryAxis=[0 0 1]  FollAlignAxisA=+X  BaseAlignAxisA=+Y  FollAlignAxisB=+Y  BaseAlignAxisB=+Z  RotationSequenceAxes=FollowerAxes  RotationSequence=XYX  RotationSequenceAngles=[0 0 0]  RotationSequenceAnglesUnits=deg  RotationMatrix=[1 0 0; 0 1 0; 0 0 1]
  Reference Frame : sm_lib/Frames and Transforms/Reference Frame
  Scope{1..5} (5 alike) : Scope
  Simulink-PS Converter Theta_J : nesl_utility/Simulink-PS Converter  PhysicalDomain=network_engine_domain  SubClassName=ps_input  LeftPortType=input  RightPortType=output  PseudoPeriodic=off  Frequencies=[]  NoiseDistribution=none  NoiseParameters=[]  Unit=rad  AffineConversion=off  FilteringAndDerivatives=filter  SimscapeFilterOrder=2  InputFilterTimeConstant=motion_time_constant  UdotUserProvided=2
  Simulink-PS Converter Theta_Q : nesl_utility/Simulink-PS Converter  PhysicalDomain=network_engine_domain  SubClassName=ps_input  LeftPortType=input  RightPortType=output  PseudoPeriodic=off  Frequencies=[]  NoiseDistribution=none  NoiseParameters=[]  Unit=rad  AffineConversion=off  FilteringAndDerivatives=filter  SimscapeFilterOrder=2  InputFilterTimeConstant=motion_time_constant  UdotUserProvided=0
  Simulink-PS Converter Theta_T : nesl_utility/Simulink-PS Converter  PhysicalDomain=network_engine_domain  SubClassName=ps_input  LeftPortType=input  RightPortType=output  PseudoPeriodic=off  Frequencies=[]  NoiseDistribution=none  NoiseParameters=[]  Unit=rad  AffineConversion=off  FilteringAndDerivatives=filter  SimscapeFilterOrder=2  InputFilterTimeConstant=motion_time_constant  UdotUserProvided=0
  ThetaJ_out : Scope
  ThetaQ_out : Scope
  ThetaT_out : Scope
  To Workspace : ToWorkspace  VariableName=thetaQ_out  SaveFormat=Timeseries  SampleTime=-1
  To Workspace1 : ToWorkspace  VariableName=thetaJ_out  SaveFormat=Timeseries  SampleTime=-1
  To Workspace2 : ToWorkspace  VariableName=thetaT_out  SaveFormat=Timeseries  SampleTime=-1
  TorqueT_D : Scope
  posicao_pe_D : Subsystem
      settings: PortSchema="{\"entries\":[{\"content\":{\"sides\":[{\"content\":{\"connectorIds\":[\"LConn1\"]},\"type\":\"ConnectorPlacement.EquallySpacedRectSide\",\"uuid\":\"d1ecfdf8-7ebe-4af1-bf63-6510536b3168\"},{\"content\":{\"connectorIds\":[\"Out1\",\"Out2\"],\"side\":\"RIGHT\"},\"type\":\"ConnectorPlacement.EquallySpacedRectSide\",\"uuid\":\"ea2203bb-aad8-4cc6-b714-1d05e8985fb0\"},{\"content\":{\"connectorIds\":[\"LConn2\"],\"side\":\"TOP\"},\"type\":\"ConnectorPlacement.EquallySpacedRectSide\",\"uuid\":\"9c93785d-a169-4ae6-a4ad-27289c508aaf\"},{\"content\":{\"connectorIds\":[],\"side\":\"BOTTOM\"},\"type\":\"ConnectorPlacement.EquallySpacedRectSide\",\"uuid\":\"d7c83b6a-5ba5-4db1-aa38-20581d0d21dd\"}]},\"type\":\"ConnectorPlacement.EquallySpacedConnector\",\"uuid\":\"0aa9c047-7b9e-44d9-9c0d-089578f3a65a\"}],\"packageUris\":[\"http://schema.mathworks.com/mf0/Connector/19700101\"],\"version\":\"1.0\"}"
  "Conexao D " : PMIOPort  Side=Left
  Ground : PMIOPort  Port=2  Side=Left
  BPD : PMIOPort  Port=3  Side=Left
  "Torques_JuntasD " : Outport  VectorParamsAs1DForOutWhenUnconnected=off
  Fcont_D : Outport  Port=2
  pos_peD : Outport  Port=3
  vel_peD : Outport  Port=4
  wires:
  Ang_R/1 -> Demux/1
  Demux/1 -> Simulink-PS Converter Theta_Q/1  "Theta_Q"
  Demux/3 -> Simulink-PS Converter Theta_T/1  "Theta_T"
  Gain/1 -> Simulink-PS Converter Theta_J/1
  Demux/2 -> Gain/1  "Theta_J"
  PS-Simulink Converter2/1 -> TorqueT_D/1, [torT]
  [torQ] -> Mux/1
  [torJ] -> Mux/2
  [torT] -> Mux/3
  Mux/1 -> "Torques_JuntasD "/1
  PS-Simulink Converter1/1 -> Gain1/1
  Gain1/1 -> Scope2/1, [torJ]
  PS-Simulink Converter3/1 -> Gain2/1
  Gain2/1 -> To Workspace/1, ThetaQ_out/1
  PS-Simulink Converter4/1 -> Gain3/1
  Gain3/1 -> To Workspace1/1, ThetaJ_out/1
  Gain4/1 -> To Workspace2/1, ThetaT_out/1
  PS-Simulink Converter/1 -> Scope1/1, [torQ]
  Pe_Direito_Contato/2(Fr_D) -> Bus Creator/2, Scope4/1
  Pe_Direito_Contato/1(Fn_D) -> Bus Creator/1, Scope3/1
  Pe_Direito_Contato/3(delt_D) -> Bus Creator/3, Scope5/1
  Bus Creator/1 -> Fcont_D/1
  posicao_pe_D/1(pos_peD) -> pos_peD/1
  PS-Simulink Converter5/1 -> Gain4/1
  posicao_pe_D/2(vel_peD) -> vel_peD/1
  connections:
  PERNA/RConn1 -- PERNA COXA/LConn1 -- PERNA_PE/LConn1
  PERNA COXA/RConn1 -- JOINT JOELHO S2/RConn1
  COXA QUADRIL/RConn1 -- JOINT QUADRlL S1/RConn1
  ROTACAO S0 S1/RConn1 -- JOINT QUADRlL S1/LConn1
  COXA JOELHO/LConn1 -- COXA/RConn1 -- COXA QUADRIL/LConn1
  ROTACAO S3 S4/LConn1 -- JOINT TORNOZ S3/RConn1
  PE_PERNA/RConn1 -- ROTACAO S3 S4/RConn1
  JOINT JOELHO S2/LConn1 -- COXA JOELHO/RConn1
  ROTACAO S0 S1/LConn1 -- "Conexao D "/RConn1
  Simulink-PS Converter Theta_Q/RConn1 -- JOINT QUADRlL S1/LConn2
  Simulink-PS Converter Theta_J/RConn1 -- JOINT JOELHO S2/LConn2
  Simulink-PS Converter Theta_T/RConn1 -- JOINT TORNOZ S3/LConn2
  JOINT QUADRlL S1/RConn2 -- PS-Simulink Converter3/LConn1
  PS-Simulink Converter/LConn1 -- JOINT QUADRlL S1/RConn3
  PS-Simulink Converter1/LConn1 -- JOINT JOELHO S2/RConn3
  JOINT JOELHO S2/RConn2 -- PS-Simulink Converter4/LConn1
  PS-Simulink Converter2/LConn1 -- JOINT TORNOZ S3/RConn3
  PS-Simulink Converter5/LConn1 -- JOINT TORNOZ S3/RConn2
  PERNA_PE/RConn1 -- JOINT TORNOZ S3/LConn1
  Ground/RConn1 -- Pe_Direito_Contato/LConn1
  BPD/RConn1 -- posicao_pe_D/LConn1
  PE_PERNA/LConn1 -- Reference Frame/RConn1 -- Pe_Direito_Contato/RConn1 -- posicao_pe_D/LConn2
